simulink model "gm_DynamicCompressionModel"  (R2019a)
settings: Solver=FixedStepDiscrete  StartTime=0.0  StopTime=t_end  RelTol=1e-3
InitFcn:
  | clear;
  | %DIAGNOSTIC = 0;  %% flag to give more information as simulation proceeds such as comments & plots
  | %CALIB_DIAGNOSTIC =  0; %% flag to give more information about calibration of filterbank due to overlap between filters: Mar 2016
  | %PRESCRIPT = 1;  %% flag to plot requested versus achieved insertion gains (esp for 125-250 Hz region).
  | %ipfiledigrms = -36; %% input file RMS in dB for 65 dB SPL equivalent
  | %opfiledigrms = -36; %% output file RMS in dB for 65 dB SPL equivalent
  | %equiv_ipSPL = 65; %% simulation of signal at this level through aid`
  | X_high = 1; % Maximum input
  | ref_dB = 85; X_ref = 1; % Define a reference point in X and its dBA value
  | % re_level = 10.^(.05*(equiv_ipSPL-65)); %% scale factor at start of hearing aid, to get input to desired simulation level
  | M_bits = 5;   % decides length of tables, 2^(4+M_bits)
  | 
  | NChans = 5;
  | [chan_cfs, ~ , t_atts, t_rels] ...
  |    = InitializeCompressionSettings(NChans);
  | % AidSettings5Chans;
  | 
  | %[VALID_WAV_FILE, sig, Fs, nbits, file_rms_dB, NStreams] ...
  | %  = loadwavfile(ipfiledigrms); %%  find [Fs], performs [recalculate] externally, provided valid file found
  | % VALID_WAV_FILE = 1;
  | [newfile, newpath] = uigetfile('*.wav','Open Signal File To Process.....');
  | if isequal(newfile,0) || isequal(newpath,0)
  |     fprintf(1,'\nFile not found'); VALID_WAV_FILE = 0;
  | else
  |     [sig, Fs] = audioread(strcat(newpath,newfile));
  | end
  | 
  | 
  | %% Test input: frequency sweep
  | X_thresh = 1*10^(0.05*(0-85));
  | Amplitudes = [X_thresh, X_thresh*10, X_thresh*100, X_thresh*1000, X_thresh*10000, 1]; %, X_thresh*100000];
  | 
  | %fMin = 100; %Hz
  | %fMax = 10000; %Hz
  | %Fs = 48000; %Hz
  | Fs_system = Fs;
  | Ts = 1/Fs;
  | Ts_system = Ts;
  | %tt = (0:length(sig)-1 )./Fs;
  | tt = 0:length(sig)-1;
  | tt = tt.*Ts;
  | %deltaF = (fMax - fMin)/tt(end);
  | %X_sweep = Amplitudes'*sin(2*pi*(fMin*tt +  0.5*deltaF*tt.*tt)) ;
  | 
  | %Volume = 6;
  | %sig = X_sweep(Volume,:)';
  | %% Replacing update_channel_params with only the needed pieces
  | 
  | % opplayer  = audioplayer(sig, Fs);
  | % nbits = opplayer.bitspersample;
  | %sig = resample(sig,48000,Fs);
  | %Fs = 48000;
  | 
  | 
  | % NStreams = min(size(sig));
  | EQ_SPAN_MSEC = 6;
  | 
  | insrt_frqs = [125, 250, 500, 1000, 2000, 3000, 4000, 6000, 8000, 10000 ]; %% decimal values
  | insrt_gns = [0 3 5 10 15 20 25 30 30 30]; %% prescribed dB for 65 dB input
  | %insrt_gns = 5*ones(1,length(insrt_frqs));  %no prescription
  | ... (+82 lines)
StopFcn:
  | proc_sig = double(out.proc_sig.data(:));
  | %alignedSigs = double(out.alignedSigs.data(:));
  | %[opwav, stop_ok] = savewavfile(opfiledigrms, ipfiledigrms, proc_sig, Fs, nbits, NStreams);
  | 
  | %load('SweepSimOutput.mat')
  | %X_out_Sweep_Sim(Volume,:) = proc_sig;
  | %save('SweepSimOutput.mat', 'X_out_Sweep_Sim');
undefined symbols (not defined in the file or in its folder): delayFix, ig_eq
libraries: hdlsllib x258, simulink x192
(part 2 of 5)

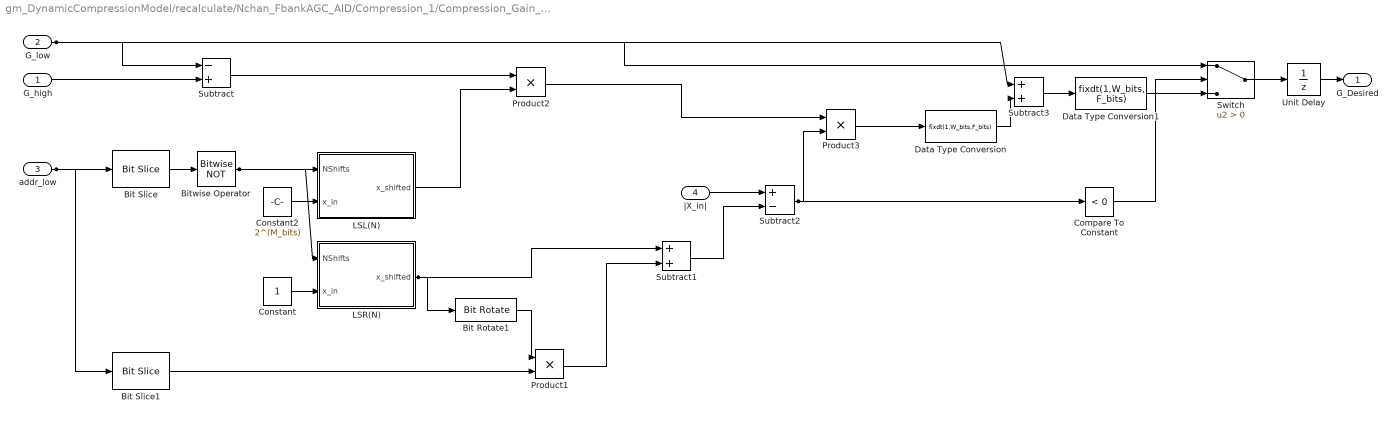
== system gm_DynamicCompressionModel/recalculate/Nchan_FbankAGC_AID/Compression_1/Compression_Gain_Calc/Linear_Approximation ==
  G_high : Inport  OutDataTypeStr=fixdt(1, 32, 28)  PortDimensions=1  SampleTime=2.08333333333333e-05
  G_low : Inport  Port=2  OutDataTypeStr=fixdt(1, 32, 28)  PortDimensions=1  SampleTime=2.08333333333333e-05
  addr_low : Inport  Port=3  OutDataTypeStr=fixdt(0, 9, 0)  PortDimensions=1  SampleTime=2.08333333333333e-05
  |X_in| : Inport  Port=4  OutDataTypeStr=fixdt(1, 32, 28)  PortDimensions=1  SampleTime=2.08333333333333e-05
  Bit Rotate1 : hdlsllib/Logic and Bit Operations/Bit Rotate  mode=Rotate Right  N=M_Bits
      settings: SourceProductName=Simulink  SourceProductBaseCode=SL
  Bit Slice : hdlsllib/Logic and Bit Operations/Bit Slice  lidx=M_Bits+3  ridx=M_Bits
      settings: SourceProductName=Simulink  SourceProductBaseCode=SL
  Bit Slice1 : hdlsllib/Logic and Bit Operations/Bit Slice  lidx=M_Bits-1  ridx=0
      settings: SourceProductName=Simulink  SourceProductBaseCode=SL
  Bitwise Operator : simulink/Logic and Bit Operations/Bitwise Operator  logicop=NOT  UseBitMask=off  BitMask=bin2dec('11011001')  BitMaskRealWorld=Stored Integer
  Compare To Constant : simulink/Logic and Bit Operations/Compare To Constant  relop=<  const=0  OutDataTypeStr=boolean
  Constant : Constant  OutDataTypeStr=fixdt(0,W_bits,W_bits-2)  SampleTime=-1
  Constant2 : Constant  Value=2^(M_bits)  OutDataTypeStr=fixdt(0,W_bits,0)  SampleTime=-1
  Data Type Conversion : DataTypeConversion  OutDataTypeStr=fixdt(1,W_bits,F_bits)
  Data Type Conversion1 : DataTypeConversion  OutDataTypeStr=fixdt(1,W_bits, F_bits)
  LSL(N) : Subsystem
  LSR(N) : Subsystem
  Product1 : Product
  Product2 : Product
  Product3 : Product
  Subtract : Sum  Inputs=-+
  Subtract1 : Sum  OutDataTypeStr=fixdt(1,W_bits, F_bits)
  Subtract2 : Sum  Inputs=+-  OutDataTypeStr=Inherit: Same as first input
  Subtract3 : Sum
  Switch : Switch  Criteria=u2 > Threshold
  Unit Delay : UnitDelay  InitialCondition=1  SampleTime=-1  HasFrameUpgradeWarning=on
  G_Desired : Outport
  wires:
  G_high/1 -> Subtract/2
  G_low/1 -> Switch/1, Subtract3/1, Subtract/1
  addr_low/1 -> Bit Slice1/1, Bit Slice/1
  |X_in|/1 -> Subtract2/1
  Bit Rotate1/1 -> Product1/1
  Bit Slice/1 -> Bitwise Operator/1
  Bit Slice1/1 -> Product1/2
  Bitwise Operator/1 -> LSR(N)/1(NShifts), LSL(N)/1(NShifts)
  Compare To Constant/1 -> Switch/2
  Constant/1 -> LSR(N)/2(x_in)
  Constant2/1 -> LSL(N)/2(x_in)
  Data Type Conversion/1 -> Subtract3/2
  Data Type Conversion1/1 -> Switch/3
  LSL(N)/1(x_shifted) -> Product2/2
  LSR(N)/1(x_shifted) -> Subtract1/1, Bit Rotate1/1
  Product1/1 -> Subtract1/2
  Product2/1 -> Product3/1
  Product3/1 -> Data Type Conversion/1
  Subtract/1 -> Product2/1
  Subtract1/1 -> Subtract2/2
  Subtract2/1 -> Product3/2, Compare To Constant/1
  Subtract3/1 -> Data Type Conversion1/1
  Switch/1 -> Unit Delay/1
  Unit Delay/1 -> G_Desired/1

== system gm_DynamicCompressionModel/recalculate/Nchan_FbankAGC_AID/Compression_1/Compression_Gain_Calc/LogAddressing ==
  note: EFFECTIVELY shift_left(x_in,NShifts)
  x_in : Inport  OutDataTypeStr=fixdt(1, 32, 28)  PortDimensions=1  SampleTime=2.08333333333333e-05
  Bit Concat : hdlsllib/Logic and Bit Operations/Bit Concat  numInputs=2
      settings: SourceProductName=Simulink
  Bit Slice : hdlsllib/Logic and Bit Operations/Bit Slice  lidx=3  ridx=0
      settings: SourceProductName=Simulink  SourceProductBaseCode=SL
  Bit Slice1 : hdlsllib/Logic and Bit Operations/Bit Slice  lidx=F_bits-1  ridx=F_bits-M_bits
      settings: SourceProductName=Simulink  SourceProductBaseCode=SL
  Bitwise Operator1 : simulink/Logic and Bit Operations/Bitwise Operator  logicop=NOT  UseBitMask=off  BitMask=bin2dec('11011001')  BitMaskRealWorld=Stored Integer
  Compare To Constant1 : simulink/Logic and Bit Operations/Compare To Constant  relop=>  const=15  OutDataTypeStr=boolean
  Constant1 : Constant  Value=W_bits-1-F_bits  OutDataTypeStr=fixdt(0,6,0)  SampleTime=-1
  Constant6 : Constant  Value=0  OutDataTypeStr=fixdt(0,9,0)  SampleTime=-1
  Data Type Conversion : DataTypeConversion  OutDataTypeStr=fixdt(0,W_bits,F_bits)
  Delay2 : Delay  DelayLength=1  SampleTime=Ts_system
  LSL(N) : Subsystem
  Subtract : Sum  Inputs=+-  OutDataTypeStr=Inherit: Same as first input
  Switch1 : Switch  Criteria=u2 ~= 0
  fxpt_lzc_W32 : Subsystem  TreatAsAtomicUnit=on
  addr_r : Outport
  wires:
  x_in/1 -> Data Type Conversion/1
  Bit Concat/1 -> Switch1/3
  Bit Slice/1 -> Bitwise Operator1/1, LSL(N)/1(NShifts)
  Bit Slice1/1 -> Bit Concat/2
  Bitwise Operator1/1 -> Bit Concat/1
  Compare To Constant1/1 -> Switch1/2
  Constant1/1 -> Subtract/2
  Constant6/1 -> Switch1/1
  Data Type Conversion/1 -> fxpt_lzc_W32/1(x_in), Delay2/1
  Delay2/1 -> LSL(N)/2(x_in)
  LSL(N)/1(x_shifted) -> Bit Slice1/1
  Subtract/1 -> Compare To Constant1/1, Bit Slice/1
  Switch1/1 -> addr_r/1
  fxpt_lzc_W32/1(lzc_out) -> Subtract/1

== system gm_DynamicCompressionModel/recalculate/Nchan_FbankAGC_AID/Compression_1/Compression_Gain_Calc/Low_Gain_Table ==
  wr_din : Inport  OutDataTypeStr=fixdt(1, 32, 28)  PortDimensions=1  SampleTime=2.08333333333333e-05
  wr_addr : Inport  Port=2  OutDataTypeStr=fixdt(0, 9, 0)  PortDimensions=1  SampleTime=2.08333333333333e-05
  wr_en : Inport  Port=3  OutDataTypeStr=boolean  PortDimensions=1  SampleTime=2.08333333333333e-05
  rd_addr : Inport  Port=4  OutDataTypeStr=fixdt(0, 9, 0)  PortDimensions=1  SampleTime=2.08333333333333e-05
  Data Type Conversion : DataTypeConversion  OutDataTypeStr=fixdt(0,16,0)
  Data Type Conversion1 : DataTypeConversion  OutDataTypeStr=fixdt(0,16,0)
  Signal Specification : SignalSpecification  OutDataTypeStr=fixdt(0,ram_size,0)  Dimensions=1
  Signal Specification1 : SignalSpecification  OutDataTypeStr=fixdt(0,ram_size,0)  Dimensions=1
  ram : UnitDelay  InitialCondition=Table_Fill(1: 2^(M_bits+4) )  SampleTime=-1  HasFrameUpgradeWarning=on
  ram_data : UnitDelay  SampleTime=-1  HasFrameUpgradeWarning=on
  select : Selector  IndexMode=Zero-based  InputPortWidth=2^ram_size  IndexOptions=Index vector (port)  Indices=[1 3]  OutputSizes=1
  switch : Switch  Criteria=u2 ~= 0
  wr_port : Assignment  IndexMode=Zero-based  IndexOptions=Index vector (port)  Indices=1  OutputSizes=[1 1]
  rd_dout : Outport
  wires:
  wr_din/1 -> wr_port/2
  wr_addr/1 -> Signal Specification/1
  wr_en/1 -> switch/2
  rd_addr/1 -> Signal Specification1/1
  Data Type Conversion/1 -> wr_port/3
  Data Type Conversion1/1 -> select/2
  Signal Specification/1 -> Data Type Conversion/1
  Signal Specification1/1 -> Data Type Conversion1/1
  ram/1 -> wr_port/1, switch/3, select/1
  ram_data/1 -> rd_dout/1
  select/1 -> ram_data/1
  switch/1 -> ram/1
  wr_port/1 -> switch/1

== system gm_DynamicCompressionModel/recalculate/Nchan_FbankAGC_AID/Compression_2/Compression_Envelope/Attack_Envelope ==
  note: ATTACK
  Curr : Inport  OutDataTypeStr=fixdt(1, 32, 28)  PortDimensions=1  SampleTime=2.08333333333333e-05
  Desired : Inport  Port=2  OutDataTypeStr=fixdt(1, 32, 28)  PortDimensions=1  SampleTime=2.08333333333333e-05
  Enable : EnablePort  OutDataTypeStr=boolean
  Product : Product  OutDataTypeStr=Inherit: Same as first input
  Subtract : Sum  Inputs=+-
  Subtract1 : Sum  OutDataTypeStr=fixdt(1,W_bits, F_bits)
  r_att(2) : Constant  Value=r_att(2)  OutDataTypeStr=fixdt(1,W_bits*2,W_bits+F_bits)  SampleTime=-1
  Gain_out : Outport  InitialOutput=0
  wires:
  Curr/1 -> Subtract/1
  Desired/1 -> Subtract1/2, Subtract/2
  Product/1 -> Subtract1/1
  Subtract/1 -> Product/2
  Subtract1/1 -> Gain_out/1
  r_att(2)/1 -> Product/1

== system gm_DynamicCompressionModel/recalculate/Nchan_FbankAGC_AID/Compression_2/Compression_Envelope/Release_Envelope ==
  note: RELEASE
  Curr : Inport  OutDataTypeStr=fixdt(1, 32, 28)  PortDimensions=1  SampleTime=2.08333333333333e-05
  Desired : Inport  Port=2  OutDataTypeStr=fixdt(1, 32, 28)  PortDimensions=1  SampleTime=2.08333333333333e-05
  Enable : EnablePort  OutDataTypeStr=boolean
  Product : Product  OutDataTypeStr=Inherit: Same as first input
  Subtract : Sum  Inputs=+-
  Subtract1 : Sum  Inputs=+-  OutDataTypeStr=Inherit: Same as first input
  r_rel(2) : Constant  Value=r_rel(2)  OutDataTypeStr=fixdt(1,W_bits*2,W_bits+F_bits)  SampleTime=-1
  Gain_out : Outport  InitialOutput=0
  wires:
  Curr/1 -> Subtract/2
  Desired/1 -> Subtract1/1, Subtract/1
  Product/1 -> Subtract1/2
  Subtract/1 -> Product/1
  Subtract1/1 -> Gain_out/1
  r_rel(2)/1 -> Product/2

== system gm_DynamicCompressionModel/recalculate/Nchan_FbankAGC_AID/Compression_2/Compression_Gain_Calc/High_Gain_Table ==
  wr_din : Inport  OutDataTypeStr=fixdt(1, 32, 28)  PortDimensions=1  SampleTime=2.08333333333333e-05
  wr_addr : Inport  Port=2  OutDataTypeStr=fixdt(0, 9, 0)  PortDimensions=1  SampleTime=2.08333333333333e-05
  wr_en : Inport  Port=3  OutDataTypeStr=boolean  PortDimensions=1  SampleTime=2.08333333333333e-05
  rd_addr : Inport  Port=4  OutDataTypeStr=fixdt(0, 9, 0)  PortDimensions=1  SampleTime=2.08333333333333e-05
  Data Type Conversion : DataTypeConversion  OutDataTypeStr=fixdt(0,16,0)
  Data Type Conversion1 : DataTypeConversion  OutDataTypeStr=fixdt(0,16,0)
  Signal Specification : SignalSpecification  OutDataTypeStr=fixdt(0,ram_size,0)  Dimensions=1
  Signal Specification1 : SignalSpecification  OutDataTypeStr=fixdt(0,ram_size,0)  Dimensions=1
  ram : UnitDelay  InitialCondition="Table_Fill(2^(M_bits+4)+1   : 2*2^(M_bits+4) )"  SampleTime=-1  HasFrameUpgradeWarning=on
  ram_data : UnitDelay  SampleTime=-1  HasFrameUpgradeWarning=on
  select : Selector  IndexMode=Zero-based  InputPortWidth=2^ram_size  IndexOptions=Index vector (port)  Indices=[1 3]  OutputSizes=1
  switch : Switch  Criteria=u2 ~= 0
  wr_port : Assignment  IndexMode=Zero-based  IndexOptions=Index vector (port)  Indices=1  OutputSizes=[1 1]
  rd_dout : Outport
  wires:
  wr_din/1 -> wr_port/2
  wr_addr/1 -> Signal Specification/1
  wr_en/1 -> switch/2
  rd_addr/1 -> Signal Specification1/1
  Data Type Conversion/1 -> wr_port/3
  Data Type Conversion1/1 -> select/2
  Signal Specification/1 -> Data Type Conversion/1
  Signal Specification1/1 -> Data Type Conversion1/1
  ram/1 -> wr_port/1, switch/3, select/1
  ram_data/1 -> rd_dout/1
  select/1 -> ram_data/1
  switch/1 -> ram/1
  wr_port/1 -> switch/1

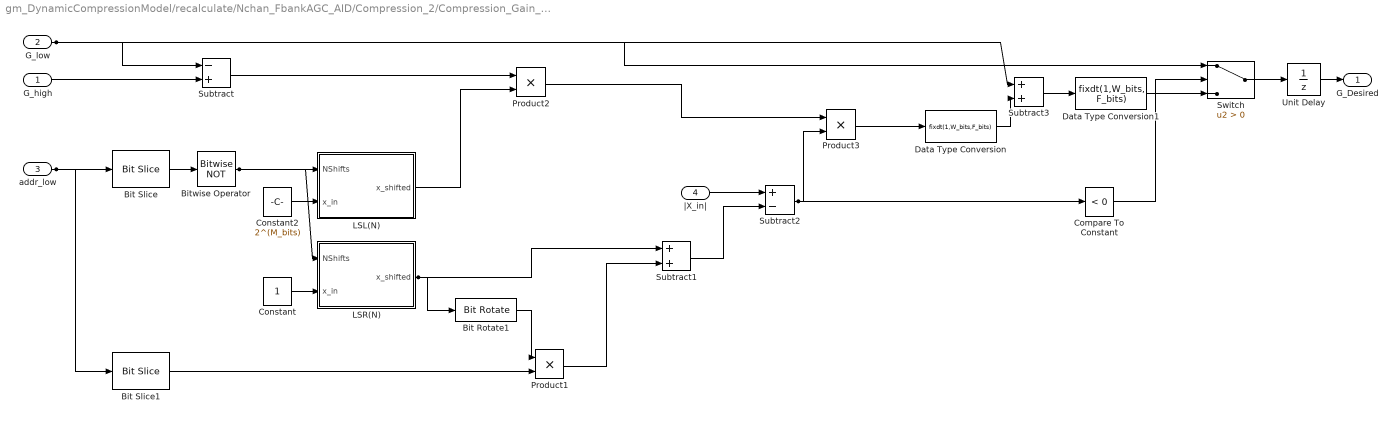
== system gm_DynamicCompressionModel/recalculate/Nchan_FbankAGC_AID/Compression_2/Compression_Gain_Calc/Linear_Approximation ==
  G_high : Inport  OutDataTypeStr=fixdt(1, 32, 28)  PortDimensions=1  SampleTime=2.08333333333333e-05
  G_low : Inport  Port=2  OutDataTypeStr=fixdt(1, 32, 28)  PortDimensions=1  SampleTime=2.08333333333333e-05
  addr_low : Inport  Port=3  OutDataTypeStr=fixdt(0, 9, 0)  PortDimensions=1  SampleTime=2.08333333333333e-05
  |X_in| : Inport  Port=4  OutDataTypeStr=fixdt(1, 32, 28)  PortDimensions=1  SampleTime=2.08333333333333e-05
  Bit Rotate1 : hdlsllib/Logic and Bit Operations/Bit Rotate  mode=Rotate Right  N=M_Bits
      settings: SourceProductName=Simulink  SourceProductBaseCode=SL
  Bit Slice : hdlsllib/Logic and Bit Operations/Bit Slice  lidx=M_Bits+3  ridx=M_Bits
      settings: SourceProductName=Simulink  SourceProductBaseCode=SL
  Bit Slice1 : hdlsllib/Logic and Bit Operations/Bit Slice  lidx=M_Bits-1  ridx=0
      settings: SourceProductName=Simulink  SourceProductBaseCode=SL
  Bitwise Operator : simulink/Logic and Bit Operations/Bitwise Operator  logicop=NOT  UseBitMask=off  BitMask=bin2dec('11011001')  BitMaskRealWorld=Stored Integer
  Compare To Constant : simulink/Logic and Bit Operations/Compare To Constant  relop=<  const=0  OutDataTypeStr=boolean
  Constant : Constant  OutDataTypeStr=fixdt(0,W_bits,W_bits-2)  SampleTime=-1
  Constant2 : Constant  Value=2^(M_bits)  OutDataTypeStr=fixdt(0,W_bits,0)  SampleTime=-1
  Data Type Conversion : DataTypeConversion  OutDataTypeStr=fixdt(1,W_bits,F_bits)
  Data Type Conversion1 : DataTypeConversion  OutDataTypeStr=fixdt(1,W_bits, F_bits)
  LSL(N) : Subsystem
  LSR(N) : Subsystem
  Product1 : Product
  Product2 : Product
  Product3 : Product
  Subtract : Sum  Inputs=-+
  Subtract1 : Sum  OutDataTypeStr=fixdt(1,W_bits, F_bits)
  Subtract2 : Sum  Inputs=+-  OutDataTypeStr=Inherit: Same as first input
  Subtract3 : Sum
  Switch : Switch  Criteria=u2 > Threshold
  Unit Delay : UnitDelay  InitialCondition=1  SampleTime=-1  HasFrameUpgradeWarning=on
  G_Desired : Outport
  wires:
  G_high/1 -> Subtract/2
  G_low/1 -> Switch/1, Subtract3/1, Subtract/1
  addr_low/1 -> Bit Slice1/1, Bit Slice/1
  |X_in|/1 -> Subtract2/1
  Bit Rotate1/1 -> Product1/1
  Bit Slice/1 -> Bitwise Operator/1
  Bit Slice1/1 -> Product1/2
  Bitwise Operator/1 -> LSR(N)/1(NShifts), LSL(N)/1(NShifts)
  Compare To Constant/1 -> Switch/2
  Constant/1 -> LSR(N)/2(x_in)
  Constant2/1 -> LSL(N)/2(x_in)
  Data Type Conversion/1 -> Subtract3/2
  Data Type Conversion1/1 -> Switch/3
  LSL(N)/1(x_shifted) -> Product2/2
  LSR(N)/1(x_shifted) -> Subtract1/1, Bit Rotate1/1
  Product1/1 -> Subtract1/2
  Product2/1 -> Product3/1
  Product3/1 -> Data Type Conversion/1
  Subtract/1 -> Product2/1
  Subtract1/1 -> Subtract2/2
  Subtract2/1 -> Product3/2, Compare To Constant/1
  Subtract3/1 -> Data Type Conversion1/1
  Switch/1 -> Unit Delay/1
  Unit Delay/1 -> G_Desired/1

== system gm_DynamicCompressionModel/recalculate/Nchan_FbankAGC_AID/Compression_2/Compression_Gain_Calc/LogAddressing ==
  note: EFFECTIVELY shift_left(x_in,NShifts)
  x_in : Inport  OutDataTypeStr=fixdt(1, 32, 28)  PortDimensions=1  SampleTime=2.08333333333333e-05
  Bit Concat : hdlsllib/Logic and Bit Operations/Bit Concat  numInputs=2
      settings: SourceProductName=Simulink
  Bit Slice : hdlsllib/Logic and Bit Operations/Bit Slice  lidx=3  ridx=0
      settings: SourceProductName=Simulink  SourceProductBaseCode=SL
  Bit Slice1 : hdlsllib/Logic and Bit Operations/Bit Slice  lidx=F_bits-1  ridx=F_bits-M_bits
      settings: SourceProductName=Simulink  SourceProductBaseCode=SL
  Bitwise Operator1 : simulink/Logic and Bit Operations/Bitwise Operator  logicop=NOT  UseBitMask=off  BitMask=bin2dec('11011001')  BitMaskRealWorld=Stored Integer
  Compare To Constant1 : simulink/Logic and Bit Operations/Compare To Constant  relop=>  const=15  OutDataTypeStr=boolean
  Constant1 : Constant  Value=W_bits-1-F_bits  OutDataTypeStr=fixdt(0,6,0)  SampleTime=-1
  Constant6 : Constant  Value=0  OutDataTypeStr=fixdt(0,9,0)  SampleTime=-1
  Data Type Conversion : DataTypeConversion  OutDataTypeStr=fixdt(0,W_bits,F_bits)
  Delay2 : Delay  DelayLength=1  SampleTime=Ts_system
  LSL(N) : Subsystem
  Subtract : Sum  Inputs=+-  OutDataTypeStr=Inherit: Same as first input
  Switch1 : Switch  Criteria=u2 ~= 0
  fxpt_lzc_W32 : Subsystem  TreatAsAtomicUnit=on
  addr_r : Outport
  wires:
  x_in/1 -> Data Type Conversion/1
  Bit Concat/1 -> Switch1/3
  Bit Slice/1 -> Bitwise Operator1/1, LSL(N)/1(NShifts)
  Bit Slice1/1 -> Bit Concat/2
  Bitwise Operator1/1 -> Bit Concat/1
  Compare To Constant1/1 -> Switch1/2
  Constant1/1 -> Subtract/2
  Constant6/1 -> Switch1/1
  Data Type Conversion/1 -> fxpt_lzc_W32/1(x_in), Delay2/1
  Delay2/1 -> LSL(N)/2(x_in)
  LSL(N)/1(x_shifted) -> Bit Slice1/1
  Subtract/1 -> Compare To Constant1/1, Bit Slice/1
  Switch1/1 -> addr_r/1
  fxpt_lzc_W32/1(lzc_out) -> Subtract/1

== system gm_DynamicCompressionModel/recalculate/Nchan_FbankAGC_AID/Compression_2/Compression_Gain_Calc/Low_Gain_Table ==
  wr_din : Inport  OutDataTypeStr=fixdt(1, 32, 28)  PortDimensions=1  SampleTime=2.08333333333333e-05
  wr_addr : Inport  Port=2  OutDataTypeStr=fixdt(0, 9, 0)  PortDimensions=1  SampleTime=2.08333333333333e-05
  wr_en : Inport  Port=3  OutDataTypeStr=boolean  PortDimensions=1  SampleTime=2.08333333333333e-05
  rd_addr : Inport  Port=4  OutDataTypeStr=fixdt(0, 9, 0)  PortDimensions=1  SampleTime=2.08333333333333e-05
  Data Type Conversion : DataTypeConversion  OutDataTypeStr=fixdt(0,16,0)
  Data Type Conversion1 : DataTypeConversion  OutDataTypeStr=fixdt(0,16,0)
  Signal Specification : SignalSpecification  OutDataTypeStr=fixdt(0,ram_size,0)  Dimensions=1
  Signal Specification1 : SignalSpecification  OutDataTypeStr=fixdt(0,ram_size,0)  Dimensions=1
  ram : UnitDelay  InitialCondition="Table_Fill(2^(M_bits+4)+1   : 2*2^(M_bits+4) )"  SampleTime=-1  HasFrameUpgradeWarning=on
  ram_data : UnitDelay  SampleTime=-1  HasFrameUpgradeWarning=on
  select : Selector  IndexMode=Zero-based  InputPortWidth=2^ram_size  IndexOptions=Index vector (port)  Indices=[1 3]  OutputSizes=1
  switch : Switch  Criteria=u2 ~= 0
  wr_port : Assignment  IndexMode=Zero-based  IndexOptions=Index vector (port)  Indices=1  OutputSizes=[1 1]
  rd_dout : Outport
  wires:
  wr_din/1 -> wr_port/2
  wr_addr/1 -> Signal Specification/1
  wr_en/1 -> switch/2
  rd_addr/1 -> Signal Specification1/1
  Data Type Conversion/1 -> wr_port/3
  Data Type Conversion1/1 -> select/2
  Signal Specification/1 -> Data Type Conversion/1
  Signal Specification1/1 -> Data Type Conversion1/1
  ram/1 -> wr_port/1, switch/3, select/1
  ram_data/1 -> rd_dout/1
  select/1 -> ram_data/1
  switch/1 -> ram/1
  wr_port/1 -> switch/1

== system gm_DynamicCompressionModel/recalculate/Nchan_FbankAGC_AID/Compression_3/Compression_Envelope/Attack_Envelope ==
  note: ATTACK
  Curr : Inport  OutDataTypeStr=fixdt(1, 32, 28)  PortDimensions=1  SampleTime=2.08333333333333e-05
  Desired : Inport  Port=2  OutDataTypeStr=fixdt(1, 32, 28)  PortDimensions=1  SampleTime=2.08333333333333e-05
  Enable : EnablePort  OutDataTypeStr=boolean
  Product : Product  OutDataTypeStr=Inherit: Same as first input
  Subtract : Sum  Inputs=+-
  Subtract1 : Sum  OutDataTypeStr=fixdt(1,W_bits, F_bits)
  r_att(3) : Constant  Value=r_att(3)  OutDataTypeStr=fixdt(1,W_bits*2,W_bits+F_bits)  SampleTime=-1
  Gain_out : Outport  InitialOutput=0
  wires:
  Curr/1 -> Subtract/1
  Desired/1 -> Subtract1/2, Subtract/2
  Product/1 -> Subtract1/1
  Subtract/1 -> Product/2
  Subtract1/1 -> Gain_out/1
  r_att(3)/1 -> Product/1

== system gm_DynamicCompressionModel/recalculate/Nchan_FbankAGC_AID/Compression_3/Compression_Envelope/Release_Envelope ==
  note: RELEASE
  Curr : Inport  OutDataTypeStr=fixdt(1, 32, 28)  PortDimensions=1  SampleTime=2.08333333333333e-05
  Desired : Inport  Port=2  OutDataTypeStr=fixdt(1, 32, 28)  PortDimensions=1  SampleTime=2.08333333333333e-05
  Enable : EnablePort  OutDataTypeStr=boolean
  Product : Product  OutDataTypeStr=Inherit: Same as first input
  Subtract : Sum  Inputs=+-
  Subtract1 : Sum  Inputs=+-  OutDataTypeStr=Inherit: Same as first input
  r_rel(3) : Constant  Value=r_rel(3)  OutDataTypeStr=fixdt(1,W_bits*2,W_bits+F_bits)  SampleTime=-1
  Gain_out : Outport  InitialOutput=0
  wires:
  Curr/1 -> Subtract/2
  Desired/1 -> Subtract1/1, Subtract/1
  Product/1 -> Subtract1/2
  Subtract/1 -> Product/1
  Subtract1/1 -> Gain_out/1
  r_rel(3)/1 -> Product/2

== system gm_DynamicCompressionModel/recalculate/Nchan_FbankAGC_AID/Compression_3/Compression_Gain_Calc/High_Gain_Table ==
  wr_din : Inport  OutDataTypeStr=fixdt(1, 32, 28)  PortDimensions=1  SampleTime=2.08333333333333e-05
  wr_addr : Inport  Port=2  OutDataTypeStr=fixdt(0, 9, 0)  PortDimensions=1  SampleTime=2.08333333333333e-05
  wr_en : Inport  Port=3  OutDataTypeStr=boolean  PortDimensions=1  SampleTime=2.08333333333333e-05
  rd_addr : Inport  Port=4  OutDataTypeStr=fixdt(0, 9, 0)  PortDimensions=1  SampleTime=2.08333333333333e-05
  Data Type Conversion : DataTypeConversion  OutDataTypeStr=fixdt(0,16,0)
  Data Type Conversion1 : DataTypeConversion  OutDataTypeStr=fixdt(0,16,0)
  Signal Specification : SignalSpecification  OutDataTypeStr=fixdt(0,ram_size,0)  Dimensions=1
  Signal Specification1 : SignalSpecification  OutDataTypeStr=fixdt(0,ram_size,0)  Dimensions=1
  ram : UnitDelay  InitialCondition=Table_Fill(2*2^(M_bits+4)+1 : 3*2^(M_bits+4) )  SampleTime=-1  HasFrameUpgradeWarning=on
  ram_data : UnitDelay  SampleTime=-1  HasFrameUpgradeWarning=on
  select : Selector  IndexMode=Zero-based  InputPortWidth=2^ram_size  IndexOptions=Index vector (port)  Indices=[1 3]  OutputSizes=1
  switch : Switch  Criteria=u2 ~= 0
  wr_port : Assignment  IndexMode=Zero-based  IndexOptions=Index vector (port)  Indices=1  OutputSizes=[1 1]
  rd_dout : Outport
  wires:
  wr_din/1 -> wr_port/2
  wr_addr/1 -> Signal Specification/1
  wr_en/1 -> switch/2
  rd_addr/1 -> Signal Specification1/1
  Data Type Conversion/1 -> wr_port/3
  Data Type Conversion1/1 -> select/2
  Signal Specification/1 -> Data Type Conversion/1
  Signal Specification1/1 -> Data Type Conversion1/1
  ram/1 -> wr_port/1, switch/3, select/1
  ram_data/1 -> rd_dout/1
  select/1 -> ram_data/1
  switch/1 -> ram/1
  wr_port/1 -> switch/1

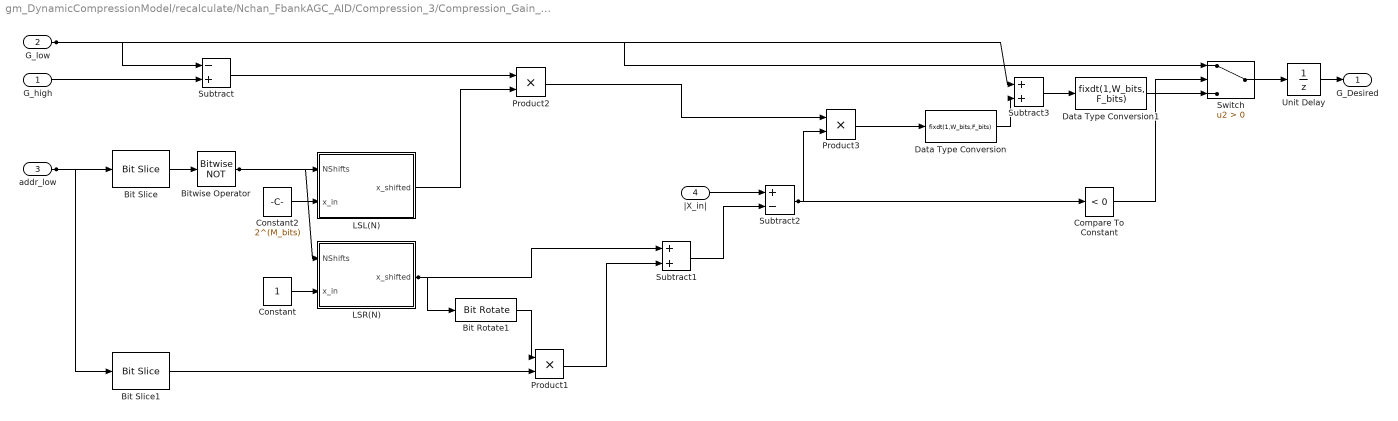
== system gm_DynamicCompressionModel/recalculate/Nchan_FbankAGC_AID/Compression_3/Compression_Gain_Calc/Linear_Approximation ==
  G_high : Inport  OutDataTypeStr=fixdt(1, 32, 28)  PortDimensions=1  SampleTime=2.08333333333333e-05
  G_low : Inport  Port=2  OutDataTypeStr=fixdt(1, 32, 28)  PortDimensions=1  SampleTime=2.08333333333333e-05
  addr_low : Inport  Port=3  OutDataTypeStr=fixdt(0, 9, 0)  PortDimensions=1  SampleTime=2.08333333333333e-05
  |X_in| : Inport  Port=4  OutDataTypeStr=fixdt(1, 32, 28)  PortDimensions=1  SampleTime=2.08333333333333e-05
  Bit Rotate1 : hdlsllib/Logic and Bit Operations/Bit Rotate  mode=Rotate Right  N=M_Bits
      settings: SourceProductName=Simulink  SourceProductBaseCode=SL
  Bit Slice : hdlsllib/Logic and Bit Operations/Bit Slice  lidx=M_Bits+3  ridx=M_Bits
      settings: SourceProductName=Simulink  SourceProductBaseCode=SL
  Bit Slice1 : hdlsllib/Logic and Bit Operations/Bit Slice  lidx=M_Bits-1  ridx=0
      settings: SourceProductName=Simulink  SourceProductBaseCode=SL
  Bitwise Operator : simulink/Logic and Bit Operations/Bitwise Operator  logicop=NOT  UseBitMask=off  BitMask=bin2dec('11011001')  BitMaskRealWorld=Stored Integer
  Compare To Constant : simulink/Logic and Bit Operations/Compare To Constant  relop=<  const=0  OutDataTypeStr=boolean
  Constant : Constant  OutDataTypeStr=fixdt(0,W_bits,W_bits-2)  SampleTime=-1
  Constant2 : Constant  Value=2^(M_bits)  OutDataTypeStr=fixdt(0,W_bits,0)  SampleTime=-1
  Data Type Conversion : DataTypeConversion  OutDataTypeStr=fixdt(1,W_bits,F_bits)
  Data Type Conversion1 : DataTypeConversion  OutDataTypeStr=fixdt(1,W_bits, F_bits)
  LSL(N) : Subsystem
  LSR(N) : Subsystem
  Product1 : Product
  Product2 : Product
  Product3 : Product
  Subtract : Sum  Inputs=-+
  Subtract1 : Sum  OutDataTypeStr=fixdt(1,W_bits, F_bits)
  Subtract2 : Sum  Inputs=+-  OutDataTypeStr=Inherit: Same as first input
  Subtract3 : Sum
  Switch : Switch  Criteria=u2 > Threshold
  Unit Delay : UnitDelay  InitialCondition=1  SampleTime=-1  HasFrameUpgradeWarning=on
  G_Desired : Outport
  wires:
  G_high/1 -> Subtract/2
  G_low/1 -> Switch/1, Subtract3/1, Subtract/1
  addr_low/1 -> Bit Slice1/1, Bit Slice/1
  |X_in|/1 -> Subtract2/1
  Bit Rotate1/1 -> Product1/1
  Bit Slice/1 -> Bitwise Operator/1
  Bit Slice1/1 -> Product1/2
  Bitwise Operator/1 -> LSR(N)/1(NShifts), LSL(N)/1(NShifts)
  Compare To Constant/1 -> Switch/2
  Constant/1 -> LSR(N)/2(x_in)
  Constant2/1 -> LSL(N)/2(x_in)
  Data Type Conversion/1 -> Subtract3/2
  Data Type Conversion1/1 -> Switch/3
  LSL(N)/1(x_shifted) -> Product2/2
  LSR(N)/1(x_shifted) -> Subtract1/1, Bit Rotate1/1
  Product1/1 -> Subtract1/2
  Product2/1 -> Product3/1
  Product3/1 -> Data Type Conversion/1
  Subtract/1 -> Product2/1
  Subtract1/1 -> Subtract2/2
  Subtract2/1 -> Product3/2, Compare To Constant/1
  Subtract3/1 -> Data Type Conversion1/1
  Switch/1 -> Unit Delay/1
  Unit Delay/1 -> G_Desired/1

== system gm_DynamicCompressionModel/recalculate/Nchan_FbankAGC_AID/Compression_3/Compression_Gain_Calc/LogAddressing ==
  note: EFFECTIVELY shift_left(x_in,NShifts)
  x_in : Inport  OutDataTypeStr=fixdt(1, 32, 28)  PortDimensions=1  SampleTime=2.08333333333333e-05
  Bit Concat : hdlsllib/Logic and Bit Operations/Bit Concat  numInputs=2
      settings: SourceProductName=Simulink
  Bit Slice : hdlsllib/Logic and Bit Operations/Bit Slice  lidx=3  ridx=0
      settings: SourceProductName=Simulink  SourceProductBaseCode=SL
  Bit Slice1 : hdlsllib/Logic and Bit Operations/Bit Slice  lidx=F_bits-1  ridx=F_bits-M_bits
      settings: SourceProductName=Simulink  SourceProductBaseCode=SL
  Bitwise Operator1 : simulink/Logic and Bit Operations/Bitwise Operator  logicop=NOT  UseBitMask=off  BitMask=bin2dec('11011001')  BitMaskRealWorld=Stored Integer
  Compare To Constant1 : simulink/Logic and Bit Operations/Compare To Constant  relop=>  const=15  OutDataTypeStr=boolean
  Constant1 : Constant  Value=W_bits-1-F_bits  OutDataTypeStr=fixdt(0,6,0)  SampleTime=-1
  Constant6 : Constant  Value=0  OutDataTypeStr=fixdt(0,9,0)  SampleTime=-1
  Data Type Conversion : DataTypeConversion  OutDataTypeStr=fixdt(0,W_bits,F_bits)
  Delay2 : Delay  DelayLength=1  SampleTime=Ts_system
  LSL(N) : Subsystem
  Subtract : Sum  Inputs=+-  OutDataTypeStr=Inherit: Same as first input
  Switch1 : Switch  Criteria=u2 ~= 0
  fxpt_lzc_W32 : Subsystem  TreatAsAtomicUnit=on
  addr_r : Outport
  wires:
  x_in/1 -> Data Type Conversion/1
  Bit Concat/1 -> Switch1/3
  Bit Slice/1 -> Bitwise Operator1/1, LSL(N)/1(NShifts)
  Bit Slice1/1 -> Bit Concat/2
  Bitwise Operator1/1 -> Bit Concat/1
  Compare To Constant1/1 -> Switch1/2
  Constant1/1 -> Subtract/2
  Constant6/1 -> Switch1/1
  Data Type Conversion/1 -> fxpt_lzc_W32/1(x_in), Delay2/1
  Delay2/1 -> LSL(N)/2(x_in)
  LSL(N)/1(x_shifted) -> Bit Slice1/1
  Subtract/1 -> Compare To Constant1/1, Bit Slice/1
  Switch1/1 -> addr_r/1
  fxpt_lzc_W32/1(lzc_out) -> Subtract/1

== system gm_DynamicCompressionModel/recalculate/Nchan_FbankAGC_AID/Compression_3/Compression_Gain_Calc/Low_Gain_Table ==
  wr_din : Inport  OutDataTypeStr=fixdt(1, 32, 28)  PortDimensions=1  SampleTime=2.08333333333333e-05
  wr_addr : Inport  Port=2  OutDataTypeStr=fixdt(0, 9, 0)  PortDimensions=1  SampleTime=2.08333333333333e-05
  wr_en : Inport  Port=3  OutDataTypeStr=boolean  PortDimensions=1  SampleTime=2.08333333333333e-05
  rd_addr : Inport  Port=4  OutDataTypeStr=fixdt(0, 9, 0)  PortDimensions=1  SampleTime=2.08333333333333e-05
  Data Type Conversion : DataTypeConversion  OutDataTypeStr=fixdt(0,16,0)
  Data Type Conversion1 : DataTypeConversion  OutDataTypeStr=fixdt(0,16,0)
  Signal Specification : SignalSpecification  OutDataTypeStr=fixdt(0,ram_size,0)  Dimensions=1
  Signal Specification1 : SignalSpecification  OutDataTypeStr=fixdt(0,ram_size,0)  Dimensions=1
  ram : UnitDelay  InitialCondition=Table_Fill(2*2^(M_bits+4)+1 : 3*2^(M_bits+4) )  SampleTime=-1  HasFrameUpgradeWarning=on
  ram_data : UnitDelay  SampleTime=-1  HasFrameUpgradeWarning=on
  select : Selector  IndexMode=Zero-based  InputPortWidth=2^ram_size  IndexOptions=Index vector (port)  Indices=[1 3]  OutputSizes=1
  switch : Switch  Criteria=u2 ~= 0
  wr_port : Assignment  IndexMode=Zero-based  IndexOptions=Index vector (port)  Indices=1  OutputSizes=[1 1]
  rd_dout : Outport
  wires:
  wr_din/1 -> wr_port/2
  wr_addr/1 -> Signal Specification/1
  wr_en/1 -> switch/2
  rd_addr/1 -> Signal Specification1/1
  Data Type Conversion/1 -> wr_port/3
  Data Type Conversion1/1 -> select/2
  Signal Specification/1 -> Data Type Conversion/1
  Signal Specification1/1 -> Data Type Conversion1/1
  ram/1 -> wr_port/1, switch/3, select/1
  ram_data/1 -> rd_dout/1
  select/1 -> ram_data/1
  switch/1 -> ram/1
  wr_port/1 -> switch/1

== system gm_DynamicCompressionModel/recalculate/Nchan_FbankAGC_AID/Compression_4/Compression_Envelope/Attack_Envelope ==
  note: ATTACK
  Curr : Inport  OutDataTypeStr=fixdt(1, 32, 28)  PortDimensions=1  SampleTime=2.08333333333333e-05
  Desired : Inport  Port=2  OutDataTypeStr=fixdt(1, 32, 28)  PortDimensions=1  SampleTime=2.08333333333333e-05
  Enable : EnablePort  OutDataTypeStr=boolean
  Product : Product  OutDataTypeStr=Inherit: Same as first input
  Subtract : Sum  Inputs=+-
  Subtract1 : Sum  OutDataTypeStr=fixdt(1,W_bits, F_bits)
  r_att(4) : Constant  Value=r_att(4)  OutDataTypeStr=fixdt(1,W_bits*2,W_bits+F_bits)  SampleTime=-1
  Gain_out : Outport  InitialOutput=0
  wires:
  Curr/1 -> Subtract/1
  Desired/1 -> Subtract1/2, Subtract/2
  Product/1 -> Subtract1/1
  Subtract/1 -> Product/2
  Subtract1/1 -> Gain_out/1
  r_att(4)/1 -> Product/1

== system gm_DynamicCompressionModel/recalculate/Nchan_FbankAGC_AID/Compression_4/Compression_Envelope/Release_Envelope ==
  note: RELEASE
  Curr : Inport  OutDataTypeStr=fixdt(1, 32, 28)  PortDimensions=1  SampleTime=2.08333333333333e-05
  Desired : Inport  Port=2  OutDataTypeStr=fixdt(1, 32, 28)  PortDimensions=1  SampleTime=2.08333333333333e-05
  Enable : EnablePort  OutDataTypeStr=boolean
  Product : Product  OutDataTypeStr=Inherit: Same as first input
  Subtract : Sum  Inputs=+-
  Subtract1 : Sum  Inputs=+-  OutDataTypeStr=Inherit: Same as first input
  r_rel(4) : Constant  Value=r_rel(4)  OutDataTypeStr=fixdt(1,W_bits*2,W_bits+F_bits)  SampleTime=-1
  Gain_out : Outport  InitialOutput=0
  wires:
  Curr/1 -> Subtract/2
  Desired/1 -> Subtract1/1, Subtract/1
  Product/1 -> Subtract1/2
  Subtract/1 -> Product/1
  Subtract1/1 -> Gain_out/1
  r_rel(4)/1 -> Product/2

== system gm_DynamicCompressionModel/recalculate/Nchan_FbankAGC_AID/Compression_4/Compression_Gain_Calc/High_Gain_Table ==
  wr_din : Inport  OutDataTypeStr=fixdt(1, 32, 28)  PortDimensions=1  SampleTime=2.08333333333333e-05
  wr_addr : Inport  Port=2  OutDataTypeStr=fixdt(0, 9, 0)  PortDimensions=1  SampleTime=2.08333333333333e-05
  wr_en : Inport  Port=3  OutDataTypeStr=boolean  PortDimensions=1  SampleTime=2.08333333333333e-05
  rd_addr : Inport  Port=4  OutDataTypeStr=fixdt(0, 9, 0)  PortDimensions=1  SampleTime=2.08333333333333e-05
  Data Type Conversion : DataTypeConversion  OutDataTypeStr=fixdt(0,16,0)
  Data Type Conversion1 : DataTypeConversion  OutDataTypeStr=fixdt(0,16,0)
  Signal Specification : SignalSpecification  OutDataTypeStr=fixdt(0,ram_size,0)  Dimensions=1
  Signal Specification1 : SignalSpecification  OutDataTypeStr=fixdt(0,ram_size,0)  Dimensions=1
  ram : UnitDelay  InitialCondition=Table_Fill(3*2^(M_bits+4)+1 : 4*2^(M_bits+4) )  SampleTime=-1  HasFrameUpgradeWarning=on
  ram_data : UnitDelay  SampleTime=-1  HasFrameUpgradeWarning=on
  select : Selector  IndexMode=Zero-based  InputPortWidth=2^ram_size  IndexOptions=Index vector (port)  Indices=[1 3]  OutputSizes=1
  switch : Switch  Criteria=u2 ~= 0
  wr_port : Assignment  IndexMode=Zero-based  IndexOptions=Index vector (port)  Indices=1  OutputSizes=[1 1]
  rd_dout : Outport
  wires:
  wr_din/1 -> wr_port/2
  wr_addr/1 -> Signal Specification/1
  wr_en/1 -> switch/2
  rd_addr/1 -> Signal Specification1/1
  Data Type Conversion/1 -> wr_port/3
  Data Type Conversion1/1 -> select/2
  Signal Specification/1 -> Data Type Conversion/1
  Signal Specification1/1 -> Data Type Conversion1/1
  ram/1 -> wr_port/1, switch/3, select/1
  ram_data/1 -> rd_dout/1
  select/1 -> ram_data/1
  switch/1 -> ram/1
  wr_port/1 -> switch/1

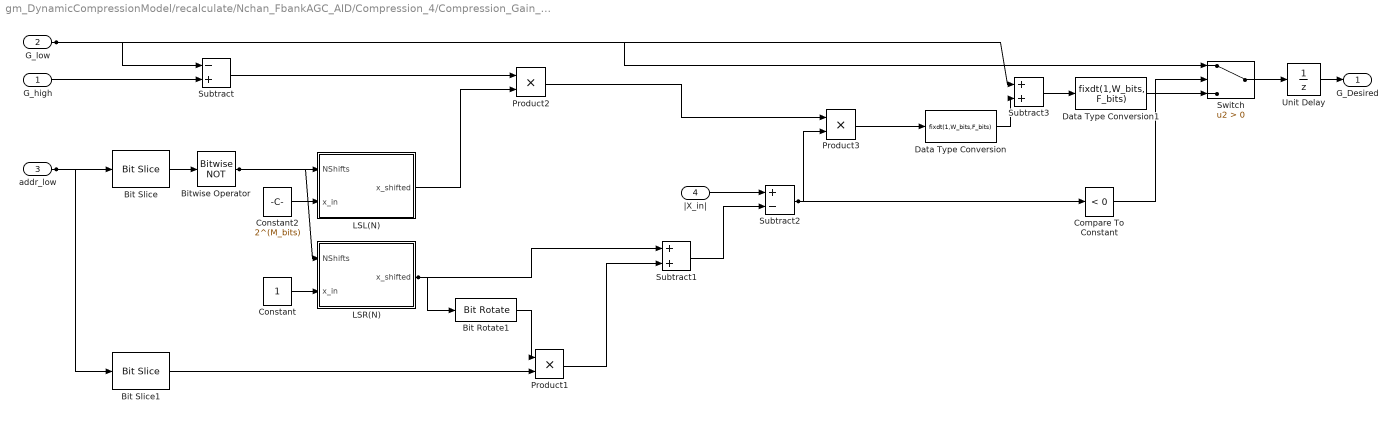
== system gm_DynamicCompressionModel/recalculate/Nchan_FbankAGC_AID/Compression_4/Compression_Gain_Calc/Linear_Approximation ==
  G_high : Inport  OutDataTypeStr=fixdt(1, 32, 28)  PortDimensions=1  SampleTime=2.08333333333333e-05
  G_low : Inport  Port=2  OutDataTypeStr=fixdt(1, 32, 28)  PortDimensions=1  SampleTime=2.08333333333333e-05
  addr_low : Inport  Port=3  OutDataTypeStr=fixdt(0, 9, 0)  PortDimensions=1  SampleTime=2.08333333333333e-05
  |X_in| : Inport  Port=4  OutDataTypeStr=fixdt(1, 32, 28)  PortDimensions=1  SampleTime=2.08333333333333e-05
  Bit Rotate1 : hdlsllib/Logic and Bit Operations/Bit Rotate  mode=Rotate Right  N=M_Bits
      settings: SourceProductName=Simulink  SourceProductBaseCode=SL
  Bit Slice : hdlsllib/Logic and Bit Operations/Bit Slice  lidx=M_Bits+3  ridx=M_Bits
      settings: SourceProductName=Simulink  SourceProductBaseCode=SL
  Bit Slice1 : hdlsllib/Logic and Bit Operations/Bit Slice  lidx=M_Bits-1  ridx=0
      settings: SourceProductName=Simulink  SourceProductBaseCode=SL
  Bitwise Operator : simulink/Logic and Bit Operations/Bitwise Operator  logicop=NOT  UseBitMask=off  BitMask=bin2dec('11011001')  BitMaskRealWorld=Stored Integer
  Compare To Constant : simulink/Logic and Bit Operations/Compare To Constant  relop=<  const=0  OutDataTypeStr=boolean
  Constant : Constant  OutDataTypeStr=fixdt(0,W_bits,W_bits-2)  SampleTime=-1
  Constant2 : Constant  Value=2^(M_bits)  OutDataTypeStr=fixdt(0,W_bits,0)  SampleTime=-1
  Data Type Conversion : DataTypeConversion  OutDataTypeStr=fixdt(1,W_bits,F_bits)
  Data Type Conversion1 : DataTypeConversion  OutDataTypeStr=fixdt(1,W_bits, F_bits)
  LSL(N) : Subsystem
  LSR(N) : Subsystem
  Product1 : Product
  Product2 : Product
  Product3 : Product
  Subtract : Sum  Inputs=-+
  Subtract1 : Sum  OutDataTypeStr=fixdt(1,W_bits, F_bits)
  Subtract2 : Sum  Inputs=+-  OutDataTypeStr=Inherit: Same as first input
  Subtract3 : Sum
  Switch : Switch  Criteria=u2 > Threshold
  Unit Delay : UnitDelay  InitialCondition=1  SampleTime=-1  HasFrameUpgradeWarning=on
  G_Desired : Outport
  wires:
  G_high/1 -> Subtract/2
  G_low/1 -> Switch/1, Subtract3/1, Subtract/1
  addr_low/1 -> Bit Slice1/1, Bit Slice/1
  |X_in|/1 -> Subtract2/1
  Bit Rotate1/1 -> Product1/1
  Bit Slice/1 -> Bitwise Operator/1
  Bit Slice1/1 -> Product1/2
  Bitwise Operator/1 -> LSR(N)/1(NShifts), LSL(N)/1(NShifts)
  Compare To Constant/1 -> Switch/2
  Constant/1 -> LSR(N)/2(x_in)
  Constant2/1 -> LSL(N)/2(x_in)
  Data Type Conversion/1 -> Subtract3/2
  Data Type Conversion1/1 -> Switch/3
  LSL(N)/1(x_shifted) -> Product2/2
  LSR(N)/1(x_shifted) -> Subtract1/1, Bit Rotate1/1
  Product1/1 -> Subtract1/2
  Product2/1 -> Product3/1
  Product3/1 -> Data Type Conversion/1
  Subtract/1 -> Product2/1
  Subtract1/1 -> Subtract2/2
  Subtract2/1 -> Product3/2, Compare To Constant/1
  Subtract3/1 -> Data Type Conversion1/1
  Switch/1 -> Unit Delay/1
  Unit Delay/1 -> G_Desired/1

== system gm_DynamicCompressionModel/recalculate/Nchan_FbankAGC_AID/Compression_4/Compression_Gain_Calc/LogAddressing ==
  note: EFFECTIVELY shift_left(x_in,NShifts)
  x_in : Inport  OutDataTypeStr=fixdt(1, 32, 28)  PortDimensions=1  SampleTime=2.08333333333333e-05
  Bit Concat : hdlsllib/Logic and Bit Operations/Bit Concat  numInputs=2
      settings: SourceProductName=Simulink
  Bit Slice : hdlsllib/Logic and Bit Operations/Bit Slice  lidx=3  ridx=0
      settings: SourceProductName=Simulink  SourceProductBaseCode=SL
  Bit Slice1 : hdlsllib/Logic and Bit Operations/Bit Slice  lidx=F_bits-1  ridx=F_bits-M_bits
      settings: SourceProductName=Simulink  SourceProductBaseCode=SL
  Bitwise Operator1 : simulink/Logic and Bit Operations/Bitwise Operator  logicop=NOT  UseBitMask=off  BitMask=bin2dec('11011001')  BitMaskRealWorld=Stored Integer
  Compare To Constant1 : simulink/Logic and Bit Operations/Compare To Constant  relop=>  const=15  OutDataTypeStr=boolean
  Constant1 : Constant  Value=W_bits-1-F_bits  OutDataTypeStr=fixdt(0,6,0)  SampleTime=-1
  Constant6 : Constant  Value=0  OutDataTypeStr=fixdt(0,9,0)  SampleTime=-1
  Data Type Conversion : DataTypeConversion  OutDataTypeStr=fixdt(0,W_bits,F_bits)
  Delay2 : Delay  DelayLength=1  SampleTime=Ts_system
  LSL(N) : Subsystem
  Subtract : Sum  Inputs=+-  OutDataTypeStr=Inherit: Same as first input
  Switch1 : Switch  Criteria=u2 ~= 0
  fxpt_lzc_W32 : Subsystem  TreatAsAtomicUnit=on
  addr_r : Outport
  wires:
  x_in/1 -> Data Type Conversion/1
  Bit Concat/1 -> Switch1/3
  Bit Slice/1 -> Bitwise Operator1/1, LSL(N)/1(NShifts)
  Bit Slice1/1 -> Bit Concat/2
  Bitwise Operator1/1 -> Bit Concat/1
  Compare To Constant1/1 -> Switch1/2
  Constant1/1 -> Subtract/2
  Constant6/1 -> Switch1/1
  Data Type Conversion/1 -> fxpt_lzc_W32/1(x_in), Delay2/1
  Delay2/1 -> LSL(N)/2(x_in)
  LSL(N)/1(x_shifted) -> Bit Slice1/1
  Subtract/1 -> Compare To Constant1/1, Bit Slice/1
  Switch1/1 -> addr_r/1
  fxpt_lzc_W32/1(lzc_out) -> Subtract/1

== system gm_DynamicCompressionModel/recalculate/Nchan_FbankAGC_AID/Compression_4/Compression_Gain_Calc/Low_Gain_Table ==
  wr_din : Inport  OutDataTypeStr=fixdt(1, 32, 28)  PortDimensions=1  SampleTime=2.08333333333333e-05
  wr_addr : Inport  Port=2  OutDataTypeStr=fixdt(0, 9, 0)  PortDimensions=1  SampleTime=2.08333333333333e-05
  wr_en : Inport  Port=3  OutDataTypeStr=boolean  PortDimensions=1  SampleTime=2.08333333333333e-05
  rd_addr : Inport  Port=4  OutDataTypeStr=fixdt(0, 9, 0)  PortDimensions=1  SampleTime=2.08333333333333e-05
  Data Type Conversion : DataTypeConversion  OutDataTypeStr=fixdt(0,16,0)
  Data Type Conversion1 : DataTypeConversion  OutDataTypeStr=fixdt(0,16,0)
  Signal Specification : SignalSpecification  OutDataTypeStr=fixdt(0,ram_size,0)  Dimensions=1
  Signal Specification1 : SignalSpecification  OutDataTypeStr=fixdt(0,ram_size,0)  Dimensions=1
  ram : UnitDelay  InitialCondition=Table_Fill(3*2^(M_bits+4)+1 : 4*2^(M_bits+4) )  SampleTime=-1  HasFrameUpgradeWarning=on
  ram_data : UnitDelay  SampleTime=-1  HasFrameUpgradeWarning=on
  select : Selector  IndexMode=Zero-based  InputPortWidth=2^ram_size  IndexOptions=Index vector (port)  Indices=[1 3]  OutputSizes=1
  switch : Switch  Criteria=u2 ~= 0
  wr_port : Assignment  IndexMode=Zero-based  IndexOptions=Index vector (port)  Indices=1  OutputSizes=[1 1]
  rd_dout : Outport
  wires:
  wr_din/1 -> wr_port/2
  wr_addr/1 -> Signal Specification/1
  wr_en/1 -> switch/2
  rd_addr/1 -> Signal Specification1/1
  Data Type Conversion/1 -> wr_port/3
  Data Type Conversion1/1 -> select/2
  Signal Specification/1 -> Data Type Conversion/1
  Signal Specification1/1 -> Data Type Conversion1/1
  ram/1 -> wr_port/1, switch/3, select/1
  ram_data/1 -> rd_dout/1
  select/1 -> ram_data/1
  switch/1 -> ram/1
  wr_port/1 -> switch/1

== system gm_DynamicCompressionModel/recalculate/Nchan_FbankAGC_AID/Compression_5/Compression_Envelope/Attack_Envelope ==
  note: ATTACK
  Curr : Inport  OutDataTypeStr=fixdt(1, 32, 28)  PortDimensions=1  SampleTime=2.08333333333333e-05
  Desired : Inport  Port=2  OutDataTypeStr=fixdt(1, 32, 28)  PortDimensions=1  SampleTime=2.08333333333333e-05
  Enable : EnablePort  OutDataTypeStr=boolean
  Product : Product  OutDataTypeStr=Inherit: Same as first input
  Subtract : Sum  Inputs=+-
  Subtract1 : Sum  OutDataTypeStr=fixdt(1,W_bits, F_bits)
  r_att(5) : Constant  Value=r_att(5)  OutDataTypeStr=fixdt(1,W_bits*2,W_bits+F_bits)  SampleTime=-1
  Gain_out : Outport  InitialOutput=0
  wires:
  Curr/1 -> Subtract/1
  Desired/1 -> Subtract1/2, Subtract/2
  Product/1 -> Subtract1/1
  Subtract/1 -> Product/2
  Subtract1/1 -> Gain_out/1
  r_att(5)/1 -> Product/1

== system gm_DynamicCompressionModel/recalculate/Nchan_FbankAGC_AID/Compression_5/Compression_Envelope/Release_Envelope ==
  note: RELEASE
  Curr : Inport  OutDataTypeStr=fixdt(1, 32, 28)  PortDimensions=1  SampleTime=2.08333333333333e-05
  Desired : Inport  Port=2  OutDataTypeStr=fixdt(1, 32, 28)  PortDimensions=1  SampleTime=2.08333333333333e-05
  Enable : EnablePort  OutDataTypeStr=boolean
  Product : Product  OutDataTypeStr=Inherit: Same as first input
  Subtract : Sum  Inputs=+-
  Subtract1 : Sum  Inputs=+-  OutDataTypeStr=Inherit: Same as first input
  r_rel(5) : Constant  Value=r_rel(5)  OutDataTypeStr=fixdt(1,W_bits*2,W_bits+F_bits)  SampleTime=-1
  Gain_out : Outport  InitialOutput=0
  wires:
  Curr/1 -> Subtract/2
  Desired/1 -> Subtract1/1, Subtract/1
  Product/1 -> Subtract1/2
  Subtract/1 -> Product/1
  Subtract1/1 -> Gain_out/1
  r_rel(5)/1 -> Product/2

== system gm_DynamicCompressionModel/recalculate/Nchan_FbankAGC_AID/Compression_5/Compression_Gain_Calc/High_Gain_Table ==
  wr_din : Inport  OutDataTypeStr=fixdt(1, 32, 28)  PortDimensions=1  SampleTime=2.08333333333333e-05
  wr_addr : Inport  Port=2  OutDataTypeStr=fixdt(0, 9, 0)  PortDimensions=1  SampleTime=2.08333333333333e-05
  wr_en : Inport  Port=3  OutDataTypeStr=boolean  PortDimensions=1  SampleTime=2.08333333333333e-05
  rd_addr : Inport  Port=4  OutDataTypeStr=fixdt(0, 9, 0)  PortDimensions=1  SampleTime=2.08333333333333e-05
  Data Type Conversion : DataTypeConversion  OutDataTypeStr=fixdt(0,16,0)
  Data Type Conversion1 : DataTypeConversion  OutDataTypeStr=fixdt(0,16,0)
  Signal Specification : SignalSpecification  OutDataTypeStr=fixdt(0,ram_size,0)  Dimensions=1
  Signal Specification1 : SignalSpecification  OutDataTypeStr=fixdt(0,ram_size,0)  Dimensions=1
  ram : UnitDelay  InitialCondition=Table_Fill(4*2^(M_bits+4)+1 : 5*2^(M_bits+4) )  SampleTime=-1  HasFrameUpgradeWarning=on
  ram_data : UnitDelay  SampleTime=-1  HasFrameUpgradeWarning=on
  select : Selector  IndexMode=Zero-based  InputPortWidth=2^ram_size  IndexOptions=Index vector (port)  Indices=[1 3]  OutputSizes=1
  switch : Switch  Criteria=u2 ~= 0
  wr_port : Assignment  IndexMode=Zero-based  IndexOptions=Index vector (port)  Indices=1  OutputSizes=[1 1]
  rd_dout : Outport
  wires:
  wr_din/1 -> wr_port/2
  wr_addr/1 -> Signal Specification/1
  wr_en/1 -> switch/2
  rd_addr/1 -> Signal Specification1/1
  Data Type Conversion/1 -> wr_port/3
  Data Type Conversion1/1 -> select/2
  Signal Specification/1 -> Data Type Conversion/1
  Signal Specification1/1 -> Data Type Conversion1/1
  ram/1 -> wr_port/1, switch/3, select/1
  ram_data/1 -> rd_dout/1
  select/1 -> ram_data/1
  switch/1 -> ram/1
  wr_port/1 -> switch/1

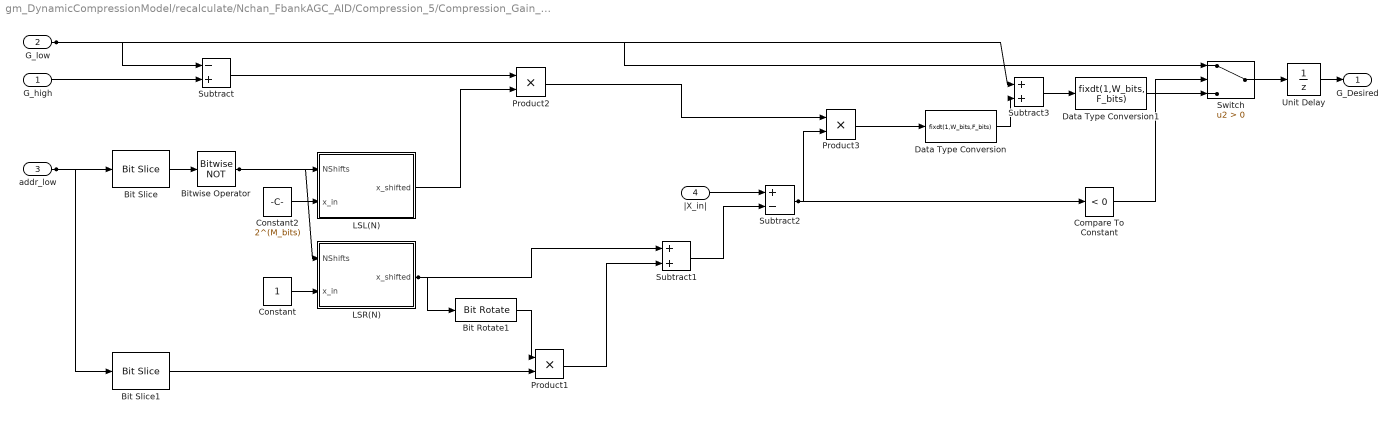
== system gm_DynamicCompressionModel/recalculate/Nchan_FbankAGC_AID/Compression_5/Compression_Gain_Calc/Linear_Approximation ==
  G_high : Inport  OutDataTypeStr=fixdt(1, 32, 28)  PortDimensions=1  SampleTime=2.08333333333333e-05
  G_low : Inport  Port=2  OutDataTypeStr=fixdt(1, 32, 28)  PortDimensions=1  SampleTime=2.08333333333333e-05
  addr_low : Inport  Port=3  OutDataTypeStr=fixdt(0, 9, 0)  PortDimensions=1  SampleTime=2.08333333333333e-05
  |X_in| : Inport  Port=4  OutDataTypeStr=fixdt(1, 32, 28)  PortDimensions=1  SampleTime=2.08333333333333e-05
  Bit Rotate1 : hdlsllib/Logic and Bit Operations/Bit Rotate  mode=Rotate Right  N=M_Bits
      settings: SourceProductName=Simulink  SourceProductBaseCode=SL
  Bit Slice : hdlsllib/Logic and Bit Operations/Bit Slice  lidx=M_Bits+3  ridx=M_Bits
      settings: SourceProductName=Simulink  SourceProductBaseCode=SL
  Bit Slice1 : hdlsllib/Logic and Bit Operations/Bit Slice  lidx=M_Bits-1  ridx=0
      settings: SourceProductName=Simulink  SourceProductBaseCode=SL
  Bitwise Operator : simulink/Logic and Bit Operations/Bitwise Operator  logicop=NOT  UseBitMask=off  BitMask=bin2dec('11011001')  BitMaskRealWorld=Stored Integer
  Compare To Constant : simulink/Logic and Bit Operations/Compare To Constant  relop=<  const=0  OutDataTypeStr=boolean
  Constant : Constant  OutDataTypeStr=fixdt(0,W_bits,W_bits-2)  SampleTime=-1
  Constant2 : Constant  Value=2^(M_bits)  OutDataTypeStr=fixdt(0,W_bits,0)  SampleTime=-1
  Data Type Conversion : DataTypeConversion  OutDataTypeStr=fixdt(1,W_bits,F_bits)
  Data Type Conversion1 : DataTypeConversion  OutDataTypeStr=fixdt(1,W_bits, F_bits)
  LSL(N) : Subsystem
  LSR(N) : Subsystem
  Product1 : Product
  Product2 : Product
  Product3 : Product
  Subtract : Sum  Inputs=-+
  Subtract1 : Sum  OutDataTypeStr=fixdt(1,W_bits, F_bits)
  Subtract2 : Sum  Inputs=+-  OutDataTypeStr=Inherit: Same as first input
  Subtract3 : Sum
  Switch : Switch  Criteria=u2 > Threshold
  Unit Delay : UnitDelay  InitialCondition=1  SampleTime=-1  HasFrameUpgradeWarning=on
  G_Desired : Outport
  wires:
  G_high/1 -> Subtract/2
  G_low/1 -> Switch/1, Subtract3/1, Subtract/1
  addr_low/1 -> Bit Slice1/1, Bit Slice/1
  |X_in|/1 -> Subtract2/1
  Bit Rotate1/1 -> Product1/1
  Bit Slice/1 -> Bitwise Operator/1
  Bit Slice1/1 -> Product1/2
  Bitwise Operator/1 -> LSR(N)/1(NShifts), LSL(N)/1(NShifts)
  Compare To Constant/1 -> Switch/2
  Constant/1 -> LSR(N)/2(x_in)
  Constant2/1 -> LSL(N)/2(x_in)
  Data Type Conversion/1 -> Subtract3/2
  Data Type Conversion1/1 -> Switch/3
  LSL(N)/1(x_shifted) -> Product2/2
  LSR(N)/1(x_shifted) -> Subtract1/1, Bit Rotate1/1
  Product1/1 -> Subtract1/2
  Product2/1 -> Product3/1
  Product3/1 -> Data Type Conversion/1
  Subtract/1 -> Product2/1
  Subtract1/1 -> Subtract2/2
  Subtract2/1 -> Product3/2, Compare To Constant/1
  Subtract3/1 -> Data Type Conversion1/1
  Switch/1 -> Unit Delay/1
  Unit Delay/1 -> G_Desired/1

== system gm_DynamicCompressionModel/recalculate/Nchan_FbankAGC_AID/Compression_5/Compression_Gain_Calc/LogAddressing ==
  note: EFFECTIVELY shift_left(x_in,NShifts)
  x_in : Inport  OutDataTypeStr=fixdt(1, 32, 28)  PortDimensions=1  SampleTime=2.08333333333333e-05
  Bit Concat : hdlsllib/Logic and Bit Operations/Bit Concat  numInputs=2
      settings: SourceProductName=Simulink
  Bit Slice : hdlsllib/Logic and Bit Operations/Bit Slice  lidx=3  ridx=0
      settings: SourceProductName=Simulink  SourceProductBaseCode=SL
  Bit Slice1 : hdlsllib/Logic and Bit Operations/Bit Slice  lidx=F_bits-1  ridx=F_bits-M_bits
      settings: SourceProductName=Simulink  SourceProductBaseCode=SL
  Bitwise Operator1 : simulink/Logic and Bit Operations/Bitwise Operator  logicop=NOT  UseBitMask=off  BitMask=bin2dec('11011001')  BitMaskRealWorld=Stored Integer
  Compare To Constant1 : simulink/Logic and Bit Operations/Compare To Constant  relop=>  const=15  OutDataTypeStr=boolean
  Constant1 : Constant  Value=W_bits-1-F_bits  OutDataTypeStr=fixdt(0,6,0)  SampleTime=-1
  Constant6 : Constant  Value=0  OutDataTypeStr=fixdt(0,9,0)  SampleTime=-1
  Data Type Conversion : DataTypeConversion  OutDataTypeStr=fixdt(0,W_bits,F_bits)
  Delay2 : Delay  DelayLength=1  SampleTime=Ts_system
  LSL(N) : Subsystem
  Subtract : Sum  Inputs=+-  OutDataTypeStr=Inherit: Same as first input
  Switch1 : Switch  Criteria=u2 ~= 0
  fxpt_lzc_W32 : Subsystem  TreatAsAtomicUnit=on
  addr_r : Outport
  wires:
  x_in/1 -> Data Type Conversion/1
  Bit Concat/1 -> Switch1/3
  Bit Slice/1 -> Bitwise Operator1/1, LSL(N)/1(NShifts)
  Bit Slice1/1 -> Bit Concat/2
  Bitwise Operator1/1 -> Bit Concat/1
  Compare To Constant1/1 -> Switch1/2
  Constant1/1 -> Subtract/2
  Constant6/1 -> Switch1/1
  Data Type Conversion/1 -> fxpt_lzc_W32/1(x_in), Delay2/1
  Delay2/1 -> LSL(N)/2(x_in)
  LSL(N)/1(x_shifted) -> Bit Slice1/1
  Subtract/1 -> Compare To Constant1/1, Bit Slice/1
  Switch1/1 -> addr_r/1
  fxpt_lzc_W32/1(lzc_out) -> Subtract/1
